simulink model "boing_condition"  (Simulink 5.0)
settings: Solver=ode23t  StartTime=0.0  StopTime=13.0  RelTol=1e-3
PreLoadFcn:
  | setup_boing_condition
libraries: cmlib x4, simulink x1
settings Model: LastModifiedBy=ansgar  BlockReductionOpt=off  BooleanDataType=off

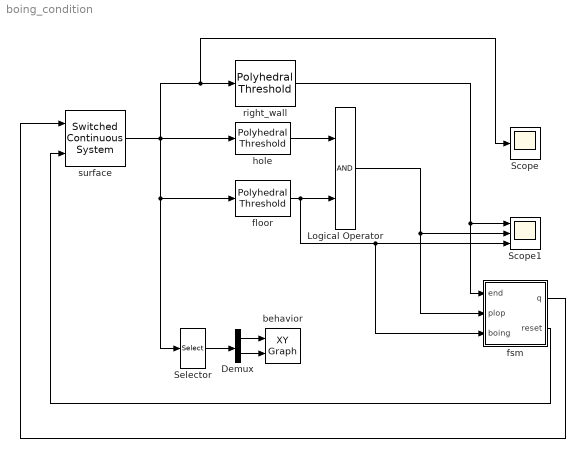
== system boing_condition ==
  Demux : Demux  Outputs=2
  Logical Operator : Logic
  Scope : Scope
  Scope1 : Scope  NumInputPorts=3
      settings: YMin=-5~-5~-5  YMax=5~5~5
  Selector : Selector  Elements=[1 2]  InputPortWidth=3
  behavior : simulink/Sinks/XY Graph  xmin=0  xmax=5  ymin=0  ymax=3  st=-1
  floor : cmlib/Polyhedral Threshold  polyhedron=floor
  fsm : Stateflow chart  TreatAsAtomicUnit=on
  hole : cmlib/Polyhedral Threshold  polyhedron=hole
  right_wall : cmlib/Polyhedral Threshold  polyhedron=right_wall
  surface : cmlib/Switched Continuous System  AncestorBlock=cmlib/Switched Continuous System  nx=3  use_sd=off  nup=[]  nz=[]  use_reset=on  nu=1  x0=[0;1+sqrt(2);0]  swfunc=boingfunc  ICS=boing_ICS  AR=boing_AR  use_param=off  p0=[]  PaCs=[]  np=0
  wires:
  fsm/2(reset) -> surface/2
  surface/1 -> hole/1, floor/1, Selector/1, right_wall/1, Scope/1
  fsm/1(q) -> surface/1
  hole/1 -> Logical Operator/1
  floor/1 -> Logical Operator/2, fsm/3(boing), Scope1/3
  Logical Operator/1 -> fsm/2(plop), Scope1/2
  Selector/1 -> Demux/1
  Demux/1 -> behavior/1
  Demux/2 -> behavior/2
  right_wall/1 -> fsm/1(end), Scope1/1

== stateflow chart fsm ==
  state idle1
    entry:q=1;
  state avoid
    entry:q=2;
  state end
    entry:q=3;
  (default) -> idle1
  idle1 -> idle1 : [boing==1]/reset;
  idle1 -> avoid : [plop==1]
  idle1 -> end : [end==1]
  data: q output double; end input boolean; plop input boolean; boing input boolean
  events: reset output EITHER_EDGE_EVENT
